simulink model "part5_a"  (R2021b)
settings: Solver=VariableStepAuto  StartTime=0.0  StopTime=20  RelTol=1e-3
settings Model: Creator=mahya  LastModifiedBy=mahya

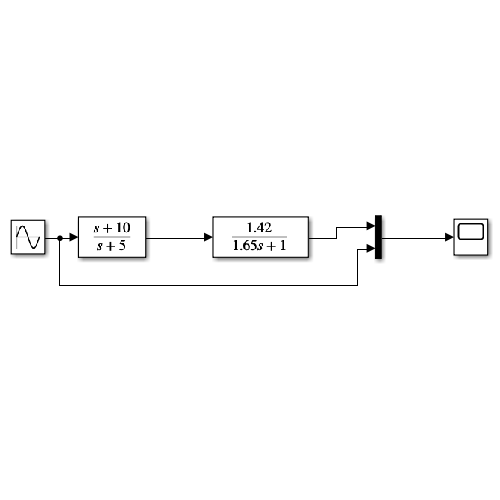
[thumbnail: Simulink's stored preview of the top-level diagram]
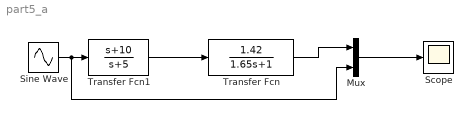
== system part5_a ==
  Mux : Mux  Inputs=2
  Scope : Scope
  Sine Wave : Sin  SampleTime=0
  Transfer Fcn : TransferFcn  Numerator=[1.42]  Denominator=[1.65 1]
  Transfer Fcn1 : TransferFcn  Numerator=[1 10]  Denominator=[1 5]
  wires:
  Transfer Fcn1/1 -> Transfer Fcn/1
  Sine Wave/1 -> Mux/2, Transfer Fcn1/1
  Mux/1 -> Scope/1
  Transfer Fcn/1 -> Mux/1
